simulink model "ChemicalProcessOptimization_PI"  (R2020a)
settings: Solver=FixedStepAuto  StartTime=0  StopTime=45  FixedStep=Ts  RelTol=1e-3  EnableMultiTasking=on
PreLoadFcn:
  | Ts = 0.5;
  | load CSTRData
values from neighbouring files (symbols this model uses):
  a_vec = [0.384207621232031;0.492686723524811;0.580956543031792;0.649017079752974;0.696868333688357;0.72451030483794;0.731942993201725;0.71916639877971;0.686180521571896;0.632985361578283;0.55958091879887;0.465967193233659;0.352144184882648;0.218111893745838;0.0638703198232284]    [run_BrainVsBench.m]    (also in run_benchmark.m)
  b_vec = [0.0628087670628903;0.0875474545057933;0.110088960048547;0.130433283691153;0.148580425433609;0.164530385275917;0.178283163218075;0.189838759260085;0.199197173401946;0.206358405643658;0.211322455985221;0.214089324426636;0.214659010967901;0.213031515609018;0.209206838349985]    [run_BrainVsBench.m]    (also in run_benchmark.m)
  conc_noise = abs(CrEQ(1)-CrEQ(5))*noise_magnitude    [init_vars.m]    (also in run_BrainVsBench.m; run_JustBrain.m; run_benchmark.m; run_brain.m)
  Cr_vec = [2 2.5 3 3.5 4 4.5 5 5.5 6 6.5 7 7.5 8 8.5 9]    [run_BrainVsBench.m]    (also in run_JustBrain.m; run_benchmark.m; run_brain.m)
  Cref_signal = 1    [init_vars.m]    (also in run_BrainVsBench.m = 2; run_JustBrain.m = 2; run_benchmark.m = 2; run_brain.m = 5)
  Ki_vec = [-7.98512854300473;-6.23612330817463;-4.75246287755465;-3.53414725114479;-2.58117642894504;-1.8935504109554;-1.47126919717588;-1.31433278760647;-1.42274118224718;-1.796494381098;-2.43559238415893;-3.34003519142998;-4.50982280291114;-5.94495521860242;-7.64543243850381]    [run_BrainVsBench.m]    (also in run_benchmark.m)
  Kp_vec = [-2.00046148741648;-2.3184560846763;-2.65393524901532;-3.00689898043353;-3.37734727893094;-3.76528014450754;-4.17069757716334;-4.59359957689834;-5.03398614371254;-5.49185727760593;-5.96721297857851;-6.4600532466303;-6.97037808176128;-7.49818748397146;-8.04348145326083]    [run_BrainVsBench.m]    (also in run_benchmark.m)
  Kt_vec = [3.60620000481947;3.57285570622906;3.55992955218359;3.56742154268306;3.59533167772747;3.64365995731683;3.71240638145112;3.80157095013036;3.91115366335453;4.04115452112365;4.19157352343771;4.36241067029671;4.55366596170065;4.76533939764953;4.99743097814336]    [run_BrainVsBench.m]    (also in run_benchmark.m)
  temp_noise = abs(TrEQ(1)-TrEQ(5))*noise_magnitude    [init_vars.m]    (also in run_BrainVsBench.m; run_JustBrain.m; run_benchmark.m; run_brain.m)
undefined symbols (not defined in the file or in its folder): CrEQ, DiscIntNeverNeededParam, sigbuilder_block, TcEQ, TrEQ
settings Model: Creator=The MathWorks, Inc.  LastModifiedBy=denisefeirstein
settings DataIOCC: InitialState=[311.267; 8.5695]  LimitDataPoints=on  SaveFormat=Array  ReturnWorkspaceOutputs=off  SignalLoggingName=logsOut
settings OptimizationCC: BooleanDataType=off  DefaultParameterBehavior=Inlined  InlineInvariantSignals=on  BufferReuse=off  ExpressionDepthLimit=2147483647  InitFltsAndDblsToZero=on  LifeSpan=inf
settings DebuggingCC: SaveWithParameterizedLinksMsg=none  UnderspecifiedInitializationDetection=Classic  MergeDetectMultiDrivingBlocksExec=none  CheckExecutionContextPreStartOutputMsg=on  CheckExecutionContextRuntimeOutputMsg=on  SignalResolutionControl=TryResolveAllWithWarning  MultiTaskDSMMsg=warning  MultiTaskCondExecSysMsg=none  AllowSymbolicDim=off  StateNameClashWarn=warning  SFUnexpectedBacktrackingDiag=warning  SFNoUnconditionalDefaultTransitionDiag=warning  SFExecutionAtInitializationDiag=none  ArithmeticOperatorsInVariantConditions=warning
settings HardwareCC: ProdBitPerPointer=32  ProdBitPerSizeT=32  ProdBitPerPtrDiffT=32  ProdLargestAtomicFloat=None  ProdIntDivRoundTo=Undefined  ProdEndianess=Unspecified  ProdWordSize=32  ProdHWDeviceType=32-bit Generic  TargetUnknown=on
settings ModelReferenceCC: PropagateSignalLabelsOutOfModel=off
settings SFSimCC: SimUseLocalCustomCode=off  CustomCodeUndefinedFunction=UseInterfaceOnly
settings RTWCC: RTWUseLocalCustomCode=off
settings CodeAppCC: StateflowObjectComments=on
settings GRTTargetCC: TargetFcnLib=ansi_tfl_tmw.mat  TargetLangStandard=C89/C90 (ANSI)  CombineOutputUpdateFcns=off  GRTInterface=on
settings ConfigComp: CovMetricSettings=dw  CovSaveCumulativeToWorkspaceVar=on  CovSaveSingleToWorkspaceVar=on  CovExternalEMLEnable=off  CovSFcnEnable=off

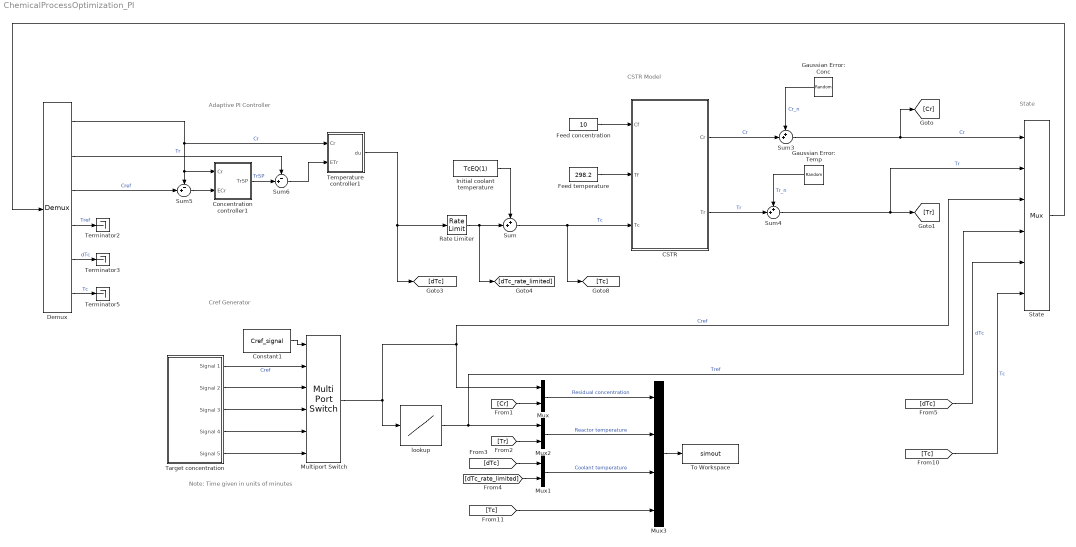
== system ChemicalProcessOptimization_PI ==
  note: Note: Time given in units of minutes
  note: Adaptive PI Controller
  note: CSTR Model
  note: Cref Generator
  note: State
  CSTR : Subsystem
  Concentration controller1 : Subsystem
  Constant1 : Constant  Value=Cref_signal
  Demux : Demux  Outputs=6
      settings: DisplayOption=none
  Feed concentration : Constant  Value=10  SampleTime=0
  Feed temperature : Constant  Value=298.2  SampleTime=0
  Gaussian Error: Conc : RandomNumber  Variance=conc_noise*conc_noise  Seed=randi(100)  SampleTime=Ts
  Gaussian Error: Temp : RandomNumber  Variance=temp_noise*temp_noise  Seed=randi(100)  SampleTime=Ts
  Initial coolant temperature : Constant  Value=TcEQ(1)  SampleTime=0
  Multiport Switch : MultiPortSwitch  Inputs=5
  Mux : Mux  Inputs=2
  Mux1 : Mux  Inputs=2
  Mux2 : Mux  Inputs=2
  Mux3 : Mux
  Rate Limiter : RateLimiter  RisingSlewLimit=10  FallingSlewLimit=-10  SampleTimeMode=inherited
  State : Mux  Inputs=6
      settings: DisplayOption=signals
  Sum : Sum  Inputs=++|
  Sum3 : Sum  Inputs=++|
  Sum4 : Sum  Inputs=++|
  Sum5 : Sum  Inputs=-+|
  Sum6 : Sum  Inputs=-+|
  Target concentration : Subsystem  Tag=STV Subsys  LoadFcn=sigbuilder_block('load',[818 356 801 540 ]);  StartFcn=sigbuilder_block('start');  StopFcn=sigbuilder_block('stop');  ClipboardFcn=sigbuilder_block('clipboard');  mask(Sigbuilder block){tuvar=[0:10]}
      mask help: Simulink:masks:SigbuilderBlock_MD
      mask init:
      | if ~strcmp(get_param(bdroot(gcbh),'SimulationStatus'),'stopped') tuvar = sigbuilder_block('maskInit'); end
      settings: CopyFcn=sigbuilder_block('copy');  DeleteFcn=sigbuilder_block('delete');  ModelCloseFcn=sigbuilder_block('modelClose');  PreSaveFcn=sigbuilder_block('preSave');  PauseFcn=sigbuilder_block('pause');  ContinueFcn=sigbuilder_block('continue');  NameChangeFcn=sigbuilder_block('namechange');  OpenFcn=sigbuilder_block('open',[991 320 801 540 ]);  CloseFcn=sigbuilder_block('close');
      mask Display: plot(0, 0, 100, 100,[2, 2, 32, 32, 2], [68, 8, 8, 68, 68],[32, 2], [38, 38], [32, 19, 2],[53, 60, 44], [32, 17, 17, 2],[16, 16, 31, 31]);txt = getActiveGroup(gcbh);text(2, 100, txt,'verticalAlignment', 'top');
  Temperature controller1 : Subsystem
  Terminator2 : Terminator
  Terminator3 : Terminator
  Terminator5 : Terminator
  To Workspace : ToWorkspace  VariableName=simout  SampleTime=-1
  lookup : Lookup_n-D  NumberOfTableDimensions=1  LookupTableObject=''  BreakpointsForDimension1=flipud(CrEQ)  Table=flipud(TrEQ)  RndMeth=Simplest  InputSameDT=on
  wires:
  Feed concentration/1 -> CSTR/1(Cf)
  Feed temperature/1 -> CSTR/2(Tf)
  Mux1/1 -> Mux3/3  "Coolant temperature"
  Initial coolant temperature/1 -> Sum/1
  [Cr] -> Mux/2
  Mux2/1 -> Mux3/2  "Reactor temperature"
  Mux/1 -> Mux3/1  "Residual concentration"
  [dTc] -> Mux1/1
  [dTc_rate_limited] -> Mux1/2
  [Tr] -> Mux2/2
  lookup/1 -> State/4, Mux2/1  "Tref"
  Sum/1 -> CSTR/3(Tc), [Tc]  "Tc"
  Mux3/1 -> To Workspace/1
  Rate Limiter/1 -> Sum/2, [dTc_rate_limited]
  Constant1/1 -> Multiport Switch/1
  Target concentration/1(Signal 1) -> Multiport Switch/2  "Cref"
  Target concentration/4(Signal 4) -> Multiport Switch/5
  Target concentration/2(Signal 2) -> Multiport Switch/3
  Target concentration/3(Signal 3) -> Multiport Switch/4
  [dTc] -> State/5  "dTc"
  CSTR/1(Cr) -> Sum3/2  "Cr"
  Gaussian Error: Conc/1 -> Sum3/1  "Cr_n"
  Gaussian Error: Temp/1 -> Sum4/1  "Tr_n"
  Temperature controller1/1(du) -> [dTc], Rate Limiter/1
  [Tc] -> State/6  "Tc"
  [Tc] -> Mux3/4
  CSTR/2(Tr) -> Sum4/2  "Tr"
  Sum3/1 -> [Cr], State/1  "Cr"
  Sum4/1 -> [Tr], State/2  "Tr"
  Multiport Switch/1 -> State/3, Mux/1, lookup/1  "Cref"
  Demux/3 -> Sum5/2  "Cref"
  Demux/1 -> Concentration controller1/1(Cr), Sum5/1, Temperature controller1/1(Cr)  "Cr"
  Demux/5 -> Terminator3/1  "dTc"
  Sum5/1 -> Concentration controller1/2(ECr)
  Demux/6 -> Terminator5/1  "Tc"
  Demux/2 -> Sum6/1  "Tr"
  Demux/4 -> Terminator2/1  "Tref"
  Concentration controller1/1(TrSP) -> Sum6/2  "TrSP"
  State/1 -> Demux/1
  Sum6/1 -> Temperature controller1/2(ETr)
  Target concentration/5(Signal 5) -> Multiport Switch/6

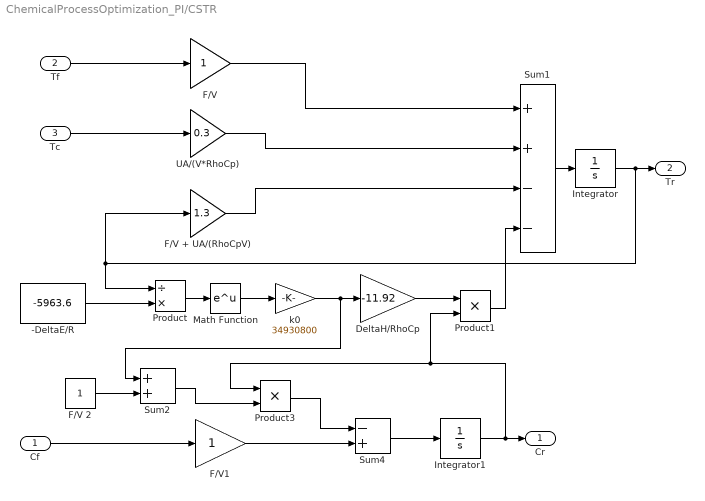
== system ChemicalProcessOptimization_PI/CSTR ==
  Cf : Inport
  Tf : Inport  Port=2
  Tc : Inport  Port=3
  -DeltaE/R : Constant  Value=-5963.6  SampleTime=0
  DeltaH/RhoCp : Gain  Gain=-11.92  SaturateOnIntegerOverflow=on  OutDataTypeStr=Inherit: Same as input  ParamDataTypeStr=Inherit: Same as input
  F/V : Gain  SaturateOnIntegerOverflow=on  OutDataTypeStr=Inherit: Same as input  ParamDataTypeStr=Inherit: Same as input
  F/V + UA/(RhoCpV) : Gain  Gain=1.3  SaturateOnIntegerOverflow=on  OutDataTypeStr=Inherit: Same as input  ParamDataTypeStr=Inherit: Same as input
  F/V 2 : Constant  SampleTime=0
  F/V1 : Gain  SaturateOnIntegerOverflow=on  OutDataTypeStr=Inherit: Same as input  ParamDataTypeStr=Inherit: Same as input
  Integrator : Integrator  InitialCondition=TrEQ(1)  LimitOutput=on  LowerSaturationLimit=0
  Integrator1 : Integrator  InitialCondition=CrEQ(1)  LimitOutput=on  LowerSaturationLimit=0
  Math Function : Math  SignedPower=on  SaturateOnIntegerOverflow=on
  Product : Product  Inputs=/*  InputSameDT=on  RndMeth=Zero  SaturateOnIntegerOverflow=on  OutDataTypeStr=Inherit: Same as first input
  Product1 : Product  InputSameDT=on  RndMeth=Zero  SaturateOnIntegerOverflow=on  OutDataTypeStr=Inherit: Same as first input
  Product3 : Product  InputSameDT=on  RndMeth=Zero  SaturateOnIntegerOverflow=on  OutDataTypeStr=Inherit: Same as first input
  Sum1 : Sum  Inputs=++--  InputSameDT=on  SaturateOnIntegerOverflow=on  OutDataTypeStr=Inherit: Same as first input
  Sum2 : Sum  InputSameDT=on  SaturateOnIntegerOverflow=on  OutDataTypeStr=Inherit: Same as first input
  Sum4 : Sum  Inputs=-+  InputSameDT=on  SaturateOnIntegerOverflow=on  OutDataTypeStr=Inherit: Same as first input
  UA/(V*RhoCp) : Gain  Gain=0.3  SaturateOnIntegerOverflow=on  OutDataTypeStr=Inherit: Same as input  ParamDataTypeStr=Inherit: Same as input
  k0 : Gain  Gain=34930800  SaturateOnIntegerOverflow=on  OutDataTypeStr=Inherit: Same as input  ParamDataTypeStr=Inherit: Same as input
  Cr : Outport
  Tr : Outport  Port=2
  wires:
  F/V/1 -> Sum1/1
  Sum1/1 -> Integrator/1
  Integrator/1 -> Product/1, F/V + UA/(RhoCpV)/1, Tr/1
  UA/(V*RhoCp)/1 -> Sum1/2
  F/V + UA/(RhoCpV)/1 -> Sum1/3
  Product/1 -> Math Function/1
  Math Function/1 -> k0/1
  DeltaH/RhoCp/1 -> Product1/1
  Product1/1 -> Sum1/4
  k0/1 -> DeltaH/RhoCp/1, Sum2/1
  -DeltaE/R/1 -> Product/2
  Product3/1 -> Sum4/1
  Sum4/1 -> Integrator1/1
  Integrator1/1 -> Product1/2, Product3/1, Cr/1
  F/V 2/1 -> Sum2/2
  F/V1/1 -> Sum4/2
  Tf/1 -> F/V/1
  Cf/1 -> F/V1/1
  Tc/1 -> UA/(V*RhoCp)/1
  Sum2/1 -> Product3/2

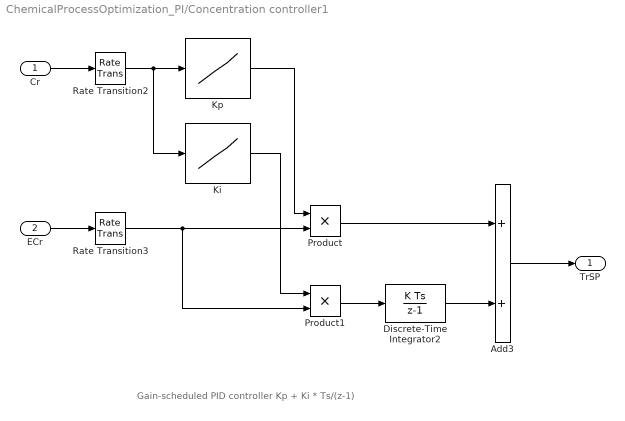
== system ChemicalProcessOptimization_PI/Concentration controller1 ==
  note: Gain-scheduled PID controller Kp + Ki * Ts/(z-1)
  Cr : Inport
  ECr : Inport  Port=2
  Add3 : Sum
  Discrete-Time Integrator2 : DiscreteIntegrator  InitialCondition=TrEQ(1)  SampleTime=Ts  ICPrevOutput=DiscIntNeverNeededParam  ICPrevScaledInput=DiscIntNeverNeededParam
  Ki : Lookup_n-D  NumberOfTableDimensions=1  LookupTableObject=''  BreakpointsForDimension1=Cr_vec  Table=Ki_vec  InternalRulePriority=Speed  RndMeth=Simplest  InputSameDT=on
  Kp : Lookup_n-D  NumberOfTableDimensions=1  LookupTableObject=''  BreakpointsForDimension1=Cr_vec  Table=Kp_vec  InternalRulePriority=Speed  RndMeth=Simplest  InputSameDT=on
  Product : Product
  Product1 : Product
  Rate Transition2 : RateTransition  OutPortSampleTime=Ts
  Rate Transition3 : RateTransition  OutPortSampleTime=Ts
  TrSP : Outport
  wires:
  ECr/1 -> Rate Transition3/1
  Discrete-Time Integrator2/1 -> Add3/2
  Product/1 -> Add3/1
  Add3/1 -> TrSP/1
  Cr/1 -> Rate Transition2/1
  Kp/1 -> Product/1
  Rate Transition2/1 -> Ki/1, Kp/1
  Product1/1 -> Discrete-Time Integrator2/1
  Rate Transition3/1 -> Product1/2, Product/2
  Ki/1 -> Product1/1

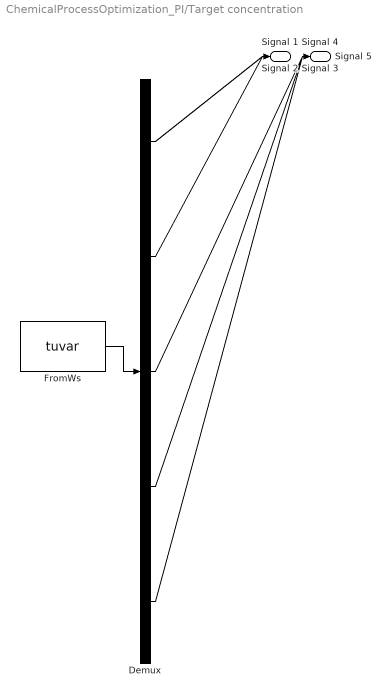
== system ChemicalProcessOptimization_PI/Target concentration ==
  Demux : Demux  Tag=STV Demux  Outputs=5
      settings: DisplayOption=none
  FromWs : FromWorkspace  Tag=STV FromWs  VariableName=tuvar
      SigBuilderData=|
      | common.afterFinalStr = 'Extrapolate'
      | common.sampleTime = 0
      | dataSet.timeRange = [0 90]
      | dataSet.name = 'Group 1'
      | sbobj.Groups.Name = 'Group 1'
      | sbobj.Groups.Signals(1).Name = 'Signal 1'
      | sbobj.Groups.Signals(1).XData = [0 10 36 90]
      | sbobj.Groups.Signals(1).YData = [8.57 8.57 2 2]
      | sbobj.Groups.Signals(2).Name = 'Signal 2'
      | sbobj.Groups.Signals(2).XData = [0 10 36 90]
      | sbobj.Groups.Signals(2).YData = [8.57 8.57 2 2]
      | sbobj.Groups.Signals(3).Name = 'Signal 3'
      | sbobj.Groups.Signals(3).XData = [0 20 46 90]
      | sbobj.Groups.Signals(3).YData = [8.57 8.57 2 2]
      | sbobj.Groups.Signals(4).Name = 'Signal 4'
      | sbobj.Groups.Signals(4).XData = [0 30 56 90]
      | sbobj.Groups.Signals(4).YData = [9.57 9.57 2 2]
      | sbobj.Groups.Signals(5).Name = 'Signal 5'
      | sbobj.Groups.Signals(5).XData = [0 90]
      | sbobj.Groups.Signals(5).YData = [8.57 8.57]
      | sbobj.Groups.TimeRange = [0 90]
  Signal 1 : Outport  Tag=STV Outport
  Signal 2 : Outport  Tag=STV Outport  Port=2
  Signal 3 : Outport  Tag=STV Outport  Port=3
  Signal 4 : Outport  Tag=STV Outport  Port=4
  Signal 5 : Outport  Tag=STV Outport  Port=5
  wires:
  FromWs/1 -> Demux/1
  Demux/1 -> Signal 1/1
  Demux/2 -> Signal 2/1
  Demux/3 -> Signal 3/1
  Demux/4 -> Signal 4/1
  Demux/5 -> Signal 5/1

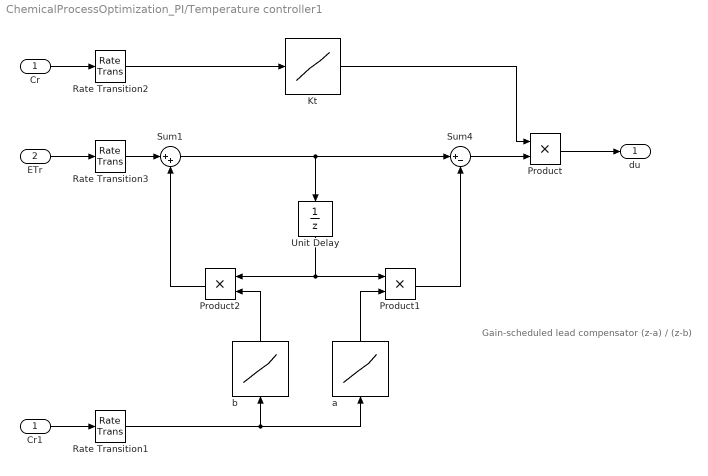
== system ChemicalProcessOptimization_PI/Temperature controller1 ==
  note: Gain-scheduled lead compensator
      | (z-a) / (z-b)
  Cr : Inport
  ETr : Inport  Port=2
  Cr1 : InportShadow
  Kt : Lookup_n-D  NumberOfTableDimensions=1  LookupTableObject=''  BreakpointsForDimension1=Cr_vec  Table=Kt_vec  InternalRulePriority=Speed  RndMeth=Simplest  InputSameDT=on
  Product : Product
  Product1 : Product
  Product2 : Product
  Rate Transition1 : RateTransition  OutPortSampleTime=Ts
  Rate Transition2 : RateTransition  OutPortSampleTime=Ts
  Rate Transition3 : RateTransition  OutPortSampleTime=Ts
  Sum1 : Sum  Inputs=|++
  Sum4 : Sum  Inputs=|+-
  Unit Delay : UnitDelay  SampleTime=Ts  HasFrameUpgradeWarning=on
  a : Lookup_n-D  NumberOfTableDimensions=1  LookupTableObject=''  BreakpointsForDimension1=Cr_vec  Table=a_vec  InternalRulePriority=Speed  RndMeth=Simplest  InputSameDT=on
  b : Lookup_n-D  NumberOfTableDimensions=1  LookupTableObject=''  BreakpointsForDimension1=Cr_vec  Table=b_vec  InternalRulePriority=Speed  RndMeth=Simplest  InputSameDT=on
  du : Outport
  wires:
  Product/1 -> du/1
  Product1/1 -> Sum4/2
  Sum1/1 -> Sum4/1, Unit Delay/1
  Sum4/1 -> Product/2
  Product2/1 -> Sum1/2
  Unit Delay/1 -> Product1/1, Product2/1
  ETr/1 -> Rate Transition3/1
  Rate Transition3/1 -> Sum1/1
  Cr/1 -> Rate Transition2/1
  Rate Transition2/1 -> Kt/1
  Kt/1 -> Product/1
  Cr1/1 -> Rate Transition1/1
  a/1 -> Product1/2
  Rate Transition1/1 -> b/1, a/1
  b/1 -> Product2/2
